simulink model "model"  (R2017a)
settings: Solver=ode4  StartTime=0.0  StopTime=100  FixedStep=0.01  MaxStep=2  MinStep=0.01  RelTol=1e-3  EnableMultiTasking=on
values from neighbouring files (symbols this model uses):
  k = 8    [Untitled.m]
  tp = 10    [Untitled.m]
undefined symbols (not defined in the file or in its folder): e0, e1, h, N, T
libraries: simulink x1
settings Model: Creator=podstawy  LastModifiedBy=Bartek
settings DataIOCC: LimitDataPoints=on  SaveFormat=Array
settings OptimizationCC: LifeSpan=inf
settings DebuggingCC: SolverPrmCheckMsg=warning  SFUnexpectedBacktrackingDiag=warning  SFNoUnconditionalDefaultTransitionDiag=warning  SFExecutionAtInitializationDiag=none
settings HardwareCC: ProdBitPerPointer=32  ProdBitPerSizeT=32  ProdBitPerPtrDiffT=32  ProdLargestAtomicFloat=None  ProdIntDivRoundTo=Undefined  ProdEndianess=Unspecified  ProdWordSize=32  ProdHWDeviceType=32-bit Generic
settings ModelReferenceCC: PropagateSignalLabelsOutOfModel=off
settings GRTTargetCC: TargetLangStandard=C89/C90 (ANSI)  GeneratePreprocessorConditionals=Disable all
settings ConfigComp: CovMetricSettings=dw  CovHtmlReporting=on  CovSaveCumulativeToWorkspaceVar=on  CovSaveSingleToWorkspaceVar=on  CovExternalEMLEnable=off  CovSFcnEnable=off

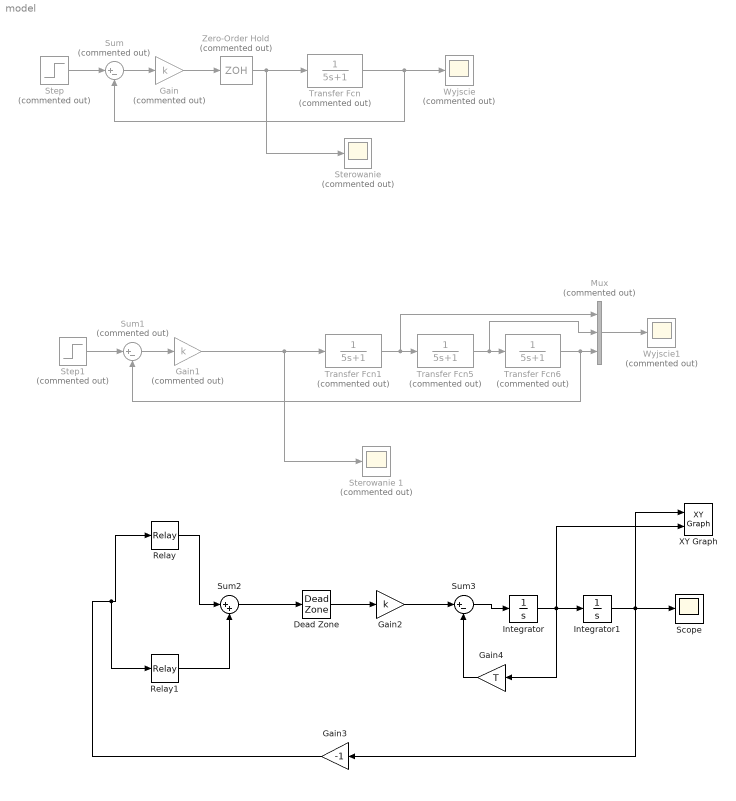
== system model ==
  Dead Zone : DeadZone  LowerValue=-N  UpperValue=N  SaturateOnIntegerOverflow=on
  Gain : Gain  Commented=on  Gain=k
  Gain1 : Gain  Commented=on  Gain=k
  Gain2 : Gain  Gain=k
  Gain3 : Gain  Gain=-1
  Gain4 : Gain  Gain=T
  Integrator : Integrator  InitialCondition=e1
  Integrator1 : Integrator  InitialCondition=e0
  Mux : Mux  Commented=on  Inputs=3
  Relay : Relay  OnSwitchValue=N+h  OffSwitchValue=N
  Relay1 : Relay  OnSwitchValue=-N  OffSwitchValue=-N-h  OnOutputValue=0  OffOutputValue=1
  Scope : Scope
  Step : Step  Commented=on  SampleTime=0
  Step1 : Step  Commented=on  SampleTime=0
  "Sterowanie " : Scope  Commented=on
  Sterowanie 1 : Scope  Commented=on
  Sum : Sum  Commented=on  Inputs=|+-
  Sum1 : Sum  Commented=on  Inputs=|+-
  Sum2 : Sum  Inputs=|++
  Sum3 : Sum  Inputs=|+-
  Transfer Fcn{,1,5..6} (4 alike) : TransferFcn  Commented=on  Denominator=[5 1]
  Wyjscie : Scope  Commented=on
  Wyjscie1 : Scope  Commented=on
  XY Graph : simulink/Sinks/XY Graph  xmin=-1  xmax=1  ymin=-1  ymax=1  st=-1
  Zero-Order Hold : ZeroOrderHold  Commented=on  SampleTime=tp
  wires:
  Gain/1 -> Zero-Order Hold/1
  Zero-Order Hold/1 -> "Sterowanie "/1, Transfer Fcn/1
  Sum/1 -> Gain/1
  Transfer Fcn/1 -> Sum/2, Wyjscie/1
  Step/1 -> Sum/1
  Gain1/1 -> Sterowanie 1/1, Transfer Fcn1/1
  Sum1/1 -> Gain1/1
  Step1/1 -> Sum1/1
  Transfer Fcn5/1 -> Mux/2, Transfer Fcn6/1
  Transfer Fcn1/1 -> Mux/1, Transfer Fcn5/1
  Transfer Fcn6/1 -> Sum1/2, Mux/3
  Mux/1 -> Wyjscie1/1
  Gain3/1 -> Relay1/1, Relay/1
  Gain4/1 -> Sum3/2
  Gain2/1 -> Sum3/1
  Relay/1 -> Sum2/1
  Dead Zone/1 -> Gain2/1
  Integrator1/1 -> XY Graph/1, Gain3/1, Scope/1
  Integrator/1 -> XY Graph/2, Gain4/1, Integrator1/1
  Sum3/1 -> Integrator/1
  Sum2/1 -> Dead Zone/1
  Relay1/1 -> Sum2/2
